simulink model "b6_formation2"  (R2021b)
settings: Solver=FixedStepAuto  StartTime=0.0  StopTime=inf  FixedStep=sampleTime  RelTol=1e-3
PreLoadFcn:
  | % Simulation parameters
  | %load exampleMap
  | 
  | % Lidar parameters
  | sensorOffset = [0,0];
  | scanAngles = -pi/2:pi/6:pi/2;
  | maxRange = 0.3;
InitFcn:
  | sampleTime = 0.05;
  | nMedianSize=3;
  | % Robot parameters
  | wheelRadius = 0.0335;
  | robotRadius = 0.8*0.116;
  | 
  | %角速度坐标
  | ks=1;
  | 
  | % Lidar parameters
  | sensorOffset = [0,0];
  | scanAngles = -pi:pi/36:pi;
  | maxRange = 0.2;
  | 
  | %车初始位置
  | init_pose_1=[1  1.3  pi/2]';
  | init_pose_2=[0.85 1  pi/2]';
  | init_pose_3=[1.15 1  pi/2]';
  | init_pose_4=[0.7  0.7 pi/2]';
  | init_pose_5=[1  0.7 pi/2]';
  | init_pose_6=[1.3 0.7  pi/2]';
  | 
  | %pp算法性能参数
  | Vd_pp=0.25;
  | Wd_pp=0.25*pi;
  | dist_pp=0.2;
  | GoalRadius=0.1;
  | numSector=72;
  | rangeDis=[0.03,maxRange];
  | thresholds=[0.03 0.1];
  | safetyDis=0.1;
  | minimumTurningRadius=0.2*0.2/3;
undefined symbols (not defined in the file): Angular, DiscIntNeverNeededParam, Linear, Pose, recovery_w, Twist
libraries: robotlib x42, dspstat3 x18, mobileRoboticsLib x7, robotmobilelib x6, robotalgslib x6
(part 4 of 5)

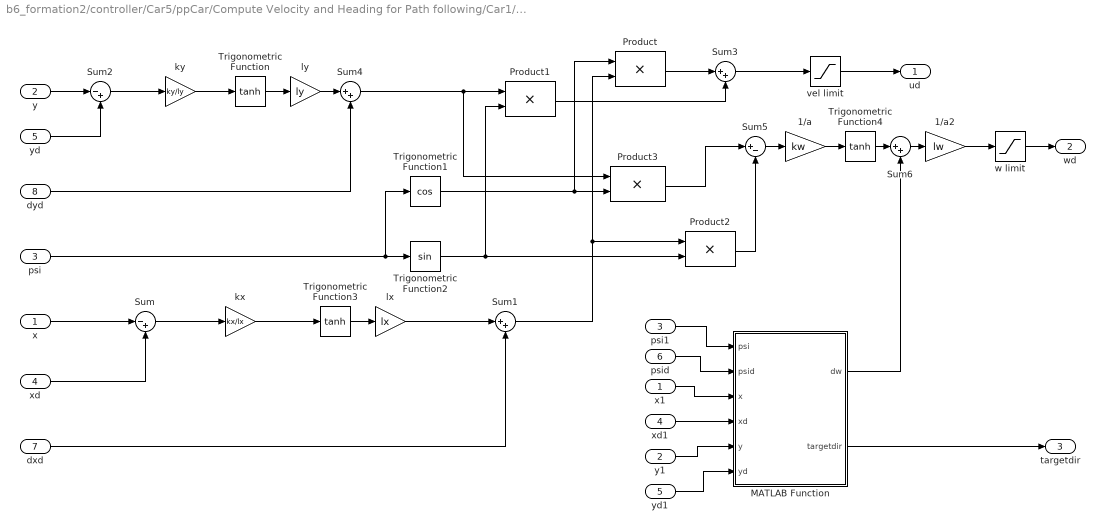
== system b6_formation2/controller/Car5/ppCar/Compute Velocity and Heading for Path following/Car1/Kinematicc Controller ==
  x : Inport
  y : Inport  Port=2
  psi : Inport  Port=3
  xd : Inport  Port=4
  yd : Inport  Port=5
  psid : Inport  Port=6
  dxd : Inport  Port=7
  dyd : Inport  Port=8
  1/a : Gain  Gain=kw  SaturateOnIntegerOverflow=on  OutDataTypeStr=Inherit: Same as input  ParamDataTypeStr=Inherit: Same as input
  1/a2 : Gain  Gain=lw  SaturateOnIntegerOverflow=on  OutDataTypeStr=Inherit: Same as input  ParamDataTypeStr=Inherit: Same as input
  MATLAB Function : MATLAB Function  TreatAsAtomicUnit=on
  Product{,1..3} (4 alike) : Product  SaturateOnIntegerOverflow=on  OutDataTypeStr=Inherit: Same as first input
  Sum : Sum  Inputs=|-+  SaturateOnIntegerOverflow=on
  Sum{1,3..4,6} (4 alike) : Sum  Inputs=|++  SaturateOnIntegerOverflow=on
  Sum2 : Sum  Inputs=|-+  SaturateOnIntegerOverflow=on
  Sum5 : Sum  Inputs=|+-  SaturateOnIntegerOverflow=on
  Trigonometric Function : Trigonometry  Operator=tanh
  Trigonometric Function1 : Trigonometry  Operator=cos
  Trigonometric Function2 : Trigonometry
  Trigonometric Function3 : Trigonometry  Operator=tanh
  Trigonometric Function4 : Trigonometry  Operator=tanh
  kx : Gain  Gain=kx/lx  SaturateOnIntegerOverflow=on  OutDataTypeStr=Inherit: Same as input  ParamDataTypeStr=Inherit: Same as input
  ky : Gain  Gain=ky/ly  SaturateOnIntegerOverflow=on  OutDataTypeStr=Inherit: Same as input  ParamDataTypeStr=Inherit: Same as input
  lx : Gain  Gain=lx  SaturateOnIntegerOverflow=on  OutDataTypeStr=Inherit: Same as input  ParamDataTypeStr=Inherit: Same as input
  ly : Gain  Gain=ly  SaturateOnIntegerOverflow=on  OutDataTypeStr=Inherit: Same as input  ParamDataTypeStr=Inherit: Same as input
  psi1 : InportShadow  Port=3
  vel limit : Saturate  UpperLimit=Vmax  LowerLimit=-0.2*Vmax
  w limit : Saturate  UpperLimit=Wmax  LowerLimit=-Wmax
  x1 : InportShadow
  xd1 : InportShadow  Port=4
  y1 : InportShadow  Port=2
  yd1 : InportShadow  Port=5
  ud : Outport
  wd : Outport  Port=2
  targetdir : Outport  Port=3
  wires:
  kx/1 -> Trigonometric Function3/1
  ky/1 -> Trigonometric Function/1
  Trigonometric Function1/1 -> Product3/2, Product/1
  Sum/1 -> kx/1
  y/1 -> Sum2/1
  Sum4/1 -> Product1/1, Product3/1
  Trigonometric Function2/1 -> Product2/2, Product1/2
  Sum3/1 -> vel limit/1
  dxd/1 -> Sum1/2
  dyd/1 -> Sum4/2
  ly/1 -> Sum4/1
  Trigonometric Function/1 -> ly/1
  lx/1 -> Sum1/1
  Trigonometric Function3/1 -> lx/1
  yd/1 -> Sum2/2
  xd/1 -> Sum/2
  x/1 -> Sum/1
  psi/1 -> Trigonometric Function2/1, Trigonometric Function1/1
  Sum1/1 -> Product2/1, Product/2
  Sum2/1 -> ky/1
  Product/1 -> Sum3/1
  Product1/1 -> Sum3/2
  Product3/1 -> Sum5/1
  Product2/1 -> Sum5/2
  Sum5/1 -> 1/a/1
  Trigonometric Function4/1 -> Sum6/1
  1/a/1 -> Trigonometric Function4/1
  vel limit/1 -> ud/1
  w limit/1 -> wd/1
  1/a2/1 -> w limit/1
  Sum6/1 -> 1/a2/1
  psid/1 -> MATLAB Function/2(psid)
  psi1/1 -> MATLAB Function/1(psi)
  x1/1 -> MATLAB Function/3(x)
  xd1/1 -> MATLAB Function/4(xd)
  y1/1 -> MATLAB Function/5(y)
  yd1/1 -> MATLAB Function/6(yd)
  MATLAB Function/1(dw) -> Sum6/2
  MATLAB Function/2(targetdir) -> targetdir/1

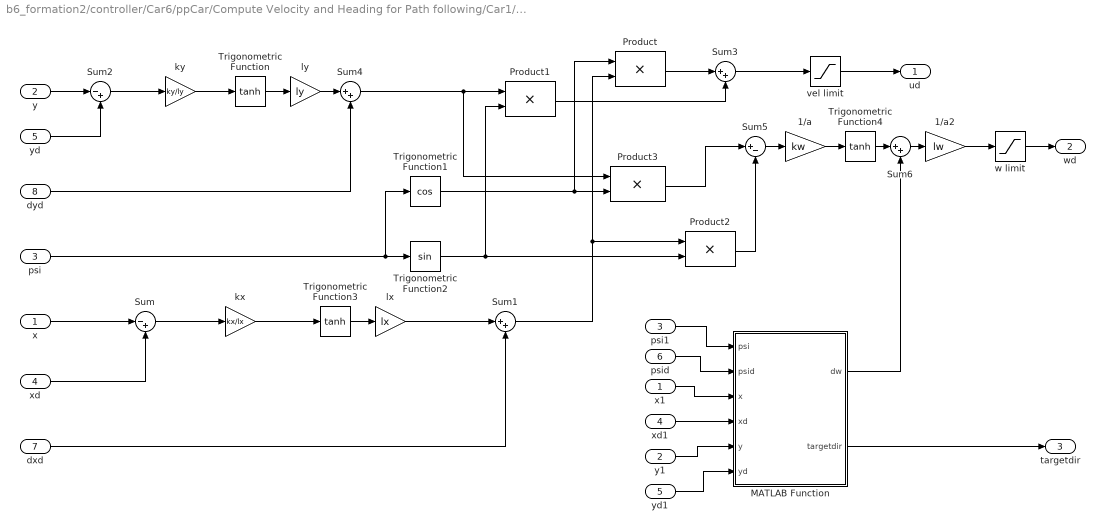
== system b6_formation2/controller/Car6/ppCar/Compute Velocity and Heading for Path following/Car1/Kinematicc Controller ==
  x : Inport
  y : Inport  Port=2
  psi : Inport  Port=3
  xd : Inport  Port=4
  yd : Inport  Port=5
  psid : Inport  Port=6
  dxd : Inport  Port=7
  dyd : Inport  Port=8
  1/a : Gain  Gain=kw  SaturateOnIntegerOverflow=on  OutDataTypeStr=Inherit: Same as input  ParamDataTypeStr=Inherit: Same as input
  1/a2 : Gain  Gain=lw  SaturateOnIntegerOverflow=on  OutDataTypeStr=Inherit: Same as input  ParamDataTypeStr=Inherit: Same as input
  MATLAB Function : MATLAB Function  TreatAsAtomicUnit=on
  Product{,1..3} (4 alike) : Product  SaturateOnIntegerOverflow=on  OutDataTypeStr=Inherit: Same as first input
  Sum : Sum  Inputs=|-+  SaturateOnIntegerOverflow=on
  Sum{1,3..4,6} (4 alike) : Sum  Inputs=|++  SaturateOnIntegerOverflow=on
  Sum2 : Sum  Inputs=|-+  SaturateOnIntegerOverflow=on
  Sum5 : Sum  Inputs=|+-  SaturateOnIntegerOverflow=on
  Trigonometric Function : Trigonometry  Operator=tanh
  Trigonometric Function1 : Trigonometry  Operator=cos
  Trigonometric Function2 : Trigonometry
  Trigonometric Function3 : Trigonometry  Operator=tanh
  Trigonometric Function4 : Trigonometry  Operator=tanh
  kx : Gain  Gain=kx/lx  SaturateOnIntegerOverflow=on  OutDataTypeStr=Inherit: Same as input  ParamDataTypeStr=Inherit: Same as input
  ky : Gain  Gain=ky/ly  SaturateOnIntegerOverflow=on  OutDataTypeStr=Inherit: Same as input  ParamDataTypeStr=Inherit: Same as input
  lx : Gain  Gain=lx  SaturateOnIntegerOverflow=on  OutDataTypeStr=Inherit: Same as input  ParamDataTypeStr=Inherit: Same as input
  ly : Gain  Gain=ly  SaturateOnIntegerOverflow=on  OutDataTypeStr=Inherit: Same as input  ParamDataTypeStr=Inherit: Same as input
  psi1 : InportShadow  Port=3
  vel limit : Saturate  UpperLimit=Vmax  LowerLimit=-0.2*Vmax
  w limit : Saturate  UpperLimit=Wmax  LowerLimit=-Wmax
  x1 : InportShadow
  xd1 : InportShadow  Port=4
  y1 : InportShadow  Port=2
  yd1 : InportShadow  Port=5
  ud : Outport
  wd : Outport  Port=2
  targetdir : Outport  Port=3
  wires:
  MATLAB Function/2(targetdir) -> targetdir/1
  MATLAB Function/1(dw) -> Sum6/2
  yd1/1 -> MATLAB Function/6(yd)
  y1/1 -> MATLAB Function/5(y)
  xd1/1 -> MATLAB Function/4(xd)
  x1/1 -> MATLAB Function/3(x)
  psi1/1 -> MATLAB Function/1(psi)
  psid/1 -> MATLAB Function/2(psid)
  Sum6/1 -> 1/a2/1
  1/a2/1 -> w limit/1
  w limit/1 -> wd/1
  vel limit/1 -> ud/1
  1/a/1 -> Trigonometric Function4/1
  Trigonometric Function4/1 -> Sum6/1
  Sum5/1 -> 1/a/1
  Product2/1 -> Sum5/2
  Product3/1 -> Sum5/1
  Product1/1 -> Sum3/2
  Product/1 -> Sum3/1
  Sum2/1 -> ky/1
  Sum1/1 -> Product/2, Product2/1
  psi/1 -> Trigonometric Function1/1, Trigonometric Function2/1
  x/1 -> Sum/1
  xd/1 -> Sum/2
  yd/1 -> Sum2/2
  Trigonometric Function3/1 -> lx/1
  lx/1 -> Sum1/1
  Trigonometric Function/1 -> ly/1
  ly/1 -> Sum4/1
  dyd/1 -> Sum4/2
  dxd/1 -> Sum1/2
  Sum3/1 -> vel limit/1
  Trigonometric Function2/1 -> Product1/2, Product2/2
  Sum4/1 -> Product3/1, Product1/1
  y/1 -> Sum2/1
  Sum/1 -> kx/1
  Trigonometric Function1/1 -> Product/1, Product3/2
  ky/1 -> Trigonometric Function/1
  kx/1 -> Trigonometric Function3/1

== matlab function b6_formation2/Subsystem/Car Pose Listener2/Subsystem/sensor2vCar4 ==
  data: V output; W output; VW_New input; VW_Msg input
function [V,W] = sensor2vCar(VW_New, VW_Msg)
persistent v0 w0
if isempty(v0)
    v0=0; 
    w0=0;    
end
if VW_New
    v0=VW_Msg.Linear.X;
    w0=VW_Msg.Angular.Z;
end

V=v0;
W=-w0;

== matlab function b6_formation2/controller/Car2/ppCar/Adjust Velocities to Avoid Obstacles/Path Following/Compute Angular Velocity ==
  data: steeringDir input; w output; wMax input
function w = exampleHelperComputeAngularVelocity(steeringDir, wMax)
%EXAMPLEHELPERCOMPUTEANGULARVELOCITY Compute angular velocity
%   W = exampleHelperComputeAngularVelocity(STEERINGDIR)
%   returns the angular velocity W for a differential drive robot in radians
%   per second for a given steering direction STEERINGDIR in the robot's
%   coordinate frame in radians.
%
%   W = exampleHelperComputeAngularVelocity(STEERINGDIR, WMAX)
%   returns the angular velocity W for a differential drive robot in radians
%   per second for a given steering direction STEERINGDIR in the robot's
%   coordinate frame in radians and maximum angular velocity WMAX in
%   radians per second. The output angular velocity is saturated based on
%   the WMAX.
%
%   Example:
%       
%       w = exampleHelperComputeAngularVelocity(0.2, 1);

% Copyright 2015 The MathWorks, Inc.

%#codegen
%#ok<*EMCA>

% Allow variable input arguments
if nargin == 1   
    wMax = inf;
end

validateattributes(steeringDir, {'double'},{'real'},...
    'exampleHelperComputeAngularVelocity', 'STEERINGDIR', 1);
validateattributes(wMax, {'double'},{'real', 'positive'},...
    'exampleHelperComputeAngularVelocity', 'WMAX', 2);

% Computing in robot's coordinate frame
curPose = [0 0 0];

% The following computation is similar to robotics.PurePursuit
lookaheadPoint = [cos(steeringDir), sin(steeringDir)];
slope = atan2((lookaheadPoint(2) - curPose(2)), ...
    (lookaheadPoint(1) - curPose(1)));
alpha = angdiff(curPose(3), slope);

% Angular velocity command for a differential drive robot is
% equal to the desired curvature to be followed by the robot.

% w = (2*sin(alpha));
% 
% % Pick a constant rotation when robot is facing in the opposite
% % direction of the path
% if abs(abs(alpha) - pi) < 1e-12
%     w = sign(w)*1;
% end
% % if abs(alpha)>pi/3
% %     w=sign(alpha)*wMax;
% % else
% %     w=0.3*alpha;
% % end
% 
% if abs(w) > wMax
%     w = sign(w)*wMax;
% end
w = sign(alpha)*wMax;

end

== matlab function b6_formation2/controller/Car2/ppCar/Compute Velocity and Heading for Path following/Car1/Kinematicc Controller/MATLAB Function ==
  data: psi input; dw output; psid input; x input; xd input; y input; yd input; targetdir output
function [dw,targetdir]= fcn(psi,psid,x,xd,y,yd)

if norm([xd-x,yd-y])<0.15    
    targetdir=angdiff(psi,psid);
    dw=tanh(targetdir);    
else
    dw=0;
    targetdir=angdiff(psi,atan2(yd-y,xd-x));
end

== matlab function b6_formation2/controller/Car1/ppCar/Adjust Velocities to Avoid Obstacles/Path Following/Compute Angular Velocity ==
  data: steeringDir input; w output; wMax input
function w = exampleHelperComputeAngularVelocity(steeringDir, wMax)
%EXAMPLEHELPERCOMPUTEANGULARVELOCITY Compute angular velocity
%   W = exampleHelperComputeAngularVelocity(STEERINGDIR)
%   returns the angular velocity W for a differential drive robot in radians
%   per second for a given steering direction STEERINGDIR in the robot's
%   coordinate frame in radians.
%
%   W = exampleHelperComputeAngularVelocity(STEERINGDIR, WMAX)
%   returns the angular velocity W for a differential drive robot in radians
%   per second for a given steering direction STEERINGDIR in the robot's
%   coordinate frame in radians and maximum angular velocity WMAX in
%   radians per second. The output angular velocity is saturated based on
%   the WMAX.
%
%   Example:
%       
%       w = exampleHelperComputeAngularVelocity(0.2, 1);

% Copyright 2015 The MathWorks, Inc.

%#codegen
%#ok<*EMCA>

% Allow variable input arguments
if nargin == 1   
    wMax = inf;
end

validateattributes(steeringDir, {'double'},{'real'},...
    'exampleHelperComputeAngularVelocity', 'STEERINGDIR', 1);
validateattributes(wMax, {'double'},{'real', 'positive'},...
    'exampleHelperComputeAngularVelocity', 'WMAX', 2);

% Computing in robot's coordinate frame
curPose = [0 0 0];

% The following computation is similar to robotics.PurePursuit
lookaheadPoint = [cos(steeringDir), sin(steeringDir)];
slope = atan2((lookaheadPoint(2) - curPose(2)), ...
    (lookaheadPoint(1) - curPose(1)));
alpha = angdiff(curPose(3), slope);

% Angular velocity command for a differential drive robot is
% equal to the desired curvature to be followed by the robot.

% w = (2*sin(alpha));
% 
% % Pick a constant rotation when robot is facing in the opposite
% % direction of the path
% if abs(abs(alpha) - pi) < 1e-12
%     w = sign(w)*1;
% end
% % if abs(alpha)>pi/3
% %     w=sign(alpha)*wMax;
% % else
% %     w=0.3*alpha;
% % end
% 
% if abs(w) > wMax
%     w = sign(w)*wMax;
% end
w = sign(alpha)*wMax;

end

== matlab function b6_formation2/controller/Car1/ppCar/Compute Velocity and Heading for Path following/Car1/Kinematicc Controller/MATLAB Function ==
  data: psi input; dw output; psid input; x input; xd input; y input; yd input; targetdir output
function [dw,targetdir]= fcn(psi,psid,x,xd,y,yd)

if norm([xd-x,yd-y])<0.15    
    targetdir=angdiff(psi,psid);
    dw=tanh(targetdir);    
else
    dw=0;
    targetdir=angdiff(psi,atan2(yd-y,xd-x));
end

== matlab function b6_formation2/ROS_simulation/ros1/MATLAB Function3 ==
  data: IsNew input; cmdMsg input; vref output; wref output
function [vref, wref] = ReadCMD(IsNew, cmdMsg)
persistent vref0 wref0
if isempty(vref0)
    vref0=0;
    wref0=0;
end
if IsNew
    vref0=cmdMsg.Linear.X;
    wref0=cmdMsg.Angular.Z;
end
vref=vref0;wref=wref0;

== matlab function b6_formation2/Subsystem/Car Pose Listener1/Subsystem/sensor2vCar ==
  data: x_init output; y_init output; yaw_init output; flag output; poseNew input; poseMsg input
function [x_init,y_init,yaw_init,flag] = sensor2vCar(poseNew, poseMsg)
persistent x0 y0 yaw0 yaw1 x0_init y0_init yaw0_init fStart
if isempty(x0)
    x0=-10; y0=-10; yaw0=0; yaw1=0;   
    x0_init=-10;y0_init=-10;yaw0_init=0;
    fStart=0;
end
if poseNew
    if x0==poseMsg.Pose.Pose.Position.X&&y0==poseMsg.Pose.Pose.Position.Y
        flag=1;
    else
        x0=poseMsg.Pose.Pose.Position.X;
        y0=poseMsg.Pose.Pose.Position.Y;   
        %yaw2=atan2(2*(poseMsg.Pose.Pose.Orientation.Z*poseMsg.Pose.Pose.Orientation.W),1-2*(poseMsg.Pose.Pose.Orientation.Z^2)); 
        eul=quat2eul([poseMsg.Pose.Pose.Orientation.W,poseMsg.Pose.Pose.Orientation.X,poseMsg.Pose.Pose.Orientation.Y,poseMsg.Pose.Pose.Orientation.Z]);
        yaw2=eul(1);
        %对前后角度差使用积分，恢复yaw的连续性
        yaw0=yaw0+angdiff(yaw1,yaw2);
        yaw1=yaw2;
        flag=0;        
        x0_init=x0;
        y0_init=y0;
        yaw0_init=yaw0;
        fStart=1;
    end 
else
    if fStart
        flag=1;
    else
        flag=0;
    end
end

x_init=x0_init;y_init=y0_init;yaw_init=yaw0_init;

== matlab function b6_formation2/controller/Car3/ppCar/Adjust Velocities to Avoid Obstacles/Path Following/Compute Angular Velocity ==
  data: steeringDir input; w output; wMax input
function w = exampleHelperComputeAngularVelocity(steeringDir, wMax)
%EXAMPLEHELPERCOMPUTEANGULARVELOCITY Compute angular velocity
%   W = exampleHelperComputeAngularVelocity(STEERINGDIR)
%   returns the angular velocity W for a differential drive robot in radians
%   per second for a given steering direction STEERINGDIR in the robot's
%   coordinate frame in radians.
%
%   W = exampleHelperComputeAngularVelocity(STEERINGDIR, WMAX)
%   returns the angular velocity W for a differential drive robot in radians
%   per second for a given steering direction STEERINGDIR in the robot's
%   coordinate frame in radians and maximum angular velocity WMAX in
%   radians per second. The output angular velocity is saturated based on
%   the WMAX.
%
%   Example:
%       
%       w = exampleHelperComputeAngularVelocity(0.2, 1);

% Copyright 2015 The MathWorks, Inc.

%#codegen
%#ok<*EMCA>

% Allow variable input arguments
if nargin == 1   
    wMax = inf;
end

validateattributes(steeringDir, {'double'},{'real'},...
    'exampleHelperComputeAngularVelocity', 'STEERINGDIR', 1);
validateattributes(wMax, {'double'},{'real', 'positive'},...
    'exampleHelperComputeAngularVelocity', 'WMAX', 2);

% Computing in robot's coordinate frame
curPose = [0 0 0];

% The following computation is similar to robotics.PurePursuit
lookaheadPoint = [cos(steeringDir), sin(steeringDir)];
slope = atan2((lookaheadPoint(2) - curPose(2)), ...
    (lookaheadPoint(1) - curPose(1)));
alpha = angdiff(curPose(3), slope);

% Angular velocity command for a differential drive robot is
% equal to the desired curvature to be followed by the robot.

% w = (2*sin(alpha));
% 
% % Pick a constant rotation when robot is facing in the opposite
% % direction of the path
% if abs(abs(alpha) - pi) < 1e-12
%     w = sign(w)*1;
% end
% % if abs(alpha)>pi/3
% %     w=sign(alpha)*wMax;
% % else
% %     w=0.3*alpha;
% % end
% 
% if abs(w) > wMax
%     w = sign(w)*wMax;
% end
w = sign(alpha)*wMax;

end

== matlab function b6_formation2/controller/Car3/ppCar/Compute Velocity and Heading for Path following/Car1/Kinematicc Controller/MATLAB Function ==
  data: psi input; dw output; psid input; x input; xd input; y input; yd input; targetdir output
function [dw,targetdir]= fcn(psi,psid,x,xd,y,yd)

if norm([xd-x,yd-y])<0.15    
    targetdir=angdiff(psi,psid);
    dw=tanh(targetdir);    
else
    dw=0;
    targetdir=angdiff(psi,atan2(yd-y,xd-x));
end

== matlab function b6_formation2/Subsystem/Car Pose Listener/Subsystem/sensor2vCar4 ==
  data: V output; W output; VW_New input; VW_Msg input
function [V,W] = sensor2vCar(VW_New, VW_Msg)
persistent v0 w0
if isempty(v0)
    v0=0; 
    w0=0;    
end
if VW_New
    v0=VW_Msg.Linear.X;
    w0=VW_Msg.Angular.Z;
end

V=v0;
W=-w0;

== matlab function b6_formation2/ROS_simulation/ros2/MATLAB Function3 ==
  data: IsNew input; cmdMsg input; vref output; wref output
function [vref, wref] = ReadCMD(IsNew, cmdMsg)
persistent vref0 wref0
if isempty(vref0)
    vref0=0;
    wref0=0;
end
if IsNew
    vref0=cmdMsg.Linear.X;
    wref0=cmdMsg.Angular.Z;
end
vref=vref0;wref=wref0;

== matlab function b6_formation2/ROS_simulation/ros3/MATLAB Function3 ==
  data: IsNew input; cmdMsg input; vref output; wref output
function [vref, wref] = ReadCMD(IsNew, cmdMsg)
persistent vref0 wref0
if isempty(vref0)
    vref0=0;
    wref0=0;
end
if IsNew
    vref0=cmdMsg.Linear.X;
    wref0=cmdMsg.Angular.Z;
end
vref=vref0;wref=wref0;

== matlab function b6_formation2/ROS_simulation/ros4/MATLAB Function3 ==
  data: IsNew input; cmdMsg input; vref output; wref output
function [vref, wref] = ReadCMD(IsNew, cmdMsg)
persistent vref0 wref0
if isempty(vref0)
    vref0=0;
    wref0=0;
end
if IsNew
    vref0=cmdMsg.Linear.X;
    wref0=cmdMsg.Angular.Z;
end
vref=vref0;wref=wref0;

== matlab function b6_formation2/controller/Car4/ppCar/Adjust Velocities to Avoid Obstacles/Path Following/Compute Angular Velocity ==
  data: steeringDir input; w output; wMax input
function w = exampleHelperComputeAngularVelocity(steeringDir, wMax)
%EXAMPLEHELPERCOMPUTEANGULARVELOCITY Compute angular velocity
%   W = exampleHelperComputeAngularVelocity(STEERINGDIR)
%   returns the angular velocity W for a differential drive robot in radians
%   per second for a given steering direction STEERINGDIR in the robot's
%   coordinate frame in radians.
%
%   W = exampleHelperComputeAngularVelocity(STEERINGDIR, WMAX)
%   returns the angular velocity W for a differential drive robot in radians
%   per second for a given steering direction STEERINGDIR in the robot's
%   coordinate frame in radians and maximum angular velocity WMAX in
%   radians per second. The output angular velocity is saturated based on
%   the WMAX.
%
%   Example:
%       
%       w = exampleHelperComputeAngularVelocity(0.2, 1);

% Copyright 2015 The MathWorks, Inc.

%#codegen
%#ok<*EMCA>

% Allow variable input arguments
if nargin == 1   
    wMax = inf;
end

validateattributes(steeringDir, {'double'},{'real'},...
    'exampleHelperComputeAngularVelocity', 'STEERINGDIR', 1);
validateattributes(wMax, {'double'},{'real', 'positive'},...
    'exampleHelperComputeAngularVelocity', 'WMAX', 2);

% Computing in robot's coordinate frame
curPose = [0 0 0];

% The following computation is similar to robotics.PurePursuit
lookaheadPoint = [cos(steeringDir), sin(steeringDir)];
slope = atan2((lookaheadPoint(2) - curPose(2)), ...
    (lookaheadPoint(1) - curPose(1)));
alpha = angdiff(curPose(3), slope);

% Angular velocity command for a differential drive robot is
% equal to the desired curvature to be followed by the robot.

% w = (2*sin(alpha));
% 
% % Pick a constant rotation when robot is facing in the opposite
% % direction of the path
% if abs(abs(alpha) - pi) < 1e-12
%     w = sign(w)*1;
% end
% % if abs(alpha)>pi/3
% %     w=sign(alpha)*wMax;
% % else
% %     w=0.3*alpha;
% % end
% 
% if abs(w) > wMax
%     w = sign(w)*wMax;
% end
w = sign(alpha)*wMax;

end

== matlab function b6_formation2/controller/Car4/ppCar/Compute Velocity and Heading for Path following/Car1/Kinematicc Controller/MATLAB Function ==
  data: psi input; dw output; psid input; x input; xd input; y input; yd input; targetdir output
function [dw,targetdir]= fcn(psi,psid,x,xd,y,yd)

if norm([xd-x,yd-y])<0.15    
    targetdir=angdiff(psi,psid);
    dw=tanh(targetdir);    
else
    dw=0;
    targetdir=angdiff(psi,atan2(yd-y,xd-x));
end

== matlab function b6_formation2/controller/Car5/ppCar/Adjust Velocities to Avoid Obstacles/Path Following/Compute Angular Velocity ==
  data: steeringDir input; w output; wMax input
function w = exampleHelperComputeAngularVelocity(steeringDir, wMax)
%EXAMPLEHELPERCOMPUTEANGULARVELOCITY Compute angular velocity
%   W = exampleHelperComputeAngularVelocity(STEERINGDIR)
%   returns the angular velocity W for a differential drive robot in radians
%   per second for a given steering direction STEERINGDIR in the robot's
%   coordinate frame in radians.
%
%   W = exampleHelperComputeAngularVelocity(STEERINGDIR, WMAX)
%   returns the angular velocity W for a differential drive robot in radians
%   per second for a given steering direction STEERINGDIR in the robot's
%   coordinate frame in radians and maximum angular velocity WMAX in
%   radians per second. The output angular velocity is saturated based on
%   the WMAX.
%
%   Example:
%       
%       w = exampleHelperComputeAngularVelocity(0.2, 1);

% Copyright 2015 The MathWorks, Inc.

%#codegen
%#ok<*EMCA>

% Allow variable input arguments
if nargin == 1   
    wMax = inf;
end

validateattributes(steeringDir, {'double'},{'real'},...
    'exampleHelperComputeAngularVelocity', 'STEERINGDIR', 1);
validateattributes(wMax, {'double'},{'real', 'positive'},...
    'exampleHelperComputeAngularVelocity', 'WMAX', 2);

% Computing in robot's coordinate frame
curPose = [0 0 0];

% The following computation is similar to robotics.PurePursuit
lookaheadPoint = [cos(steeringDir), sin(steeringDir)];
slope = atan2((lookaheadPoint(2) - curPose(2)), ...
    (lookaheadPoint(1) - curPose(1)));
alpha = angdiff(curPose(3), slope);

% Angular velocity command for a differential drive robot is
% equal to the desired curvature to be followed by the robot.

% w = (2*sin(alpha));
% 
% % Pick a constant rotation when robot is facing in the opposite
% % direction of the path
% if abs(abs(alpha) - pi) < 1e-12
%     w = sign(w)*1;
% end
% % if abs(alpha)>pi/3
% %     w=sign(alpha)*wMax;
% % else
% %     w=0.3*alpha;
% % end
% 
% if abs(w) > wMax
%     w = sign(w)*wMax;
% end
w = sign(alpha)*wMax;

end

== matlab function b6_formation2/ROS_simulation/ros1/MATLAB Function ==
  data: yaw input; x output; y output; z output; w output
function [x,y,z,w]=ToQuaternion(yaw)
%https://blog.csdn.net/xiaoma_bk/article/details/79082629
pitch=0;
roll=0;

   cy = cos(yaw * 0.5);
    sy = sin(yaw * 0.5);
    cp = cos(pitch * 0.5);
    sp = sin(pitch * 0.5);
    cr = cos(roll * 0.5);
    sr = sin(roll * 0.5);
 

   w = cy * cp * cr + sy * sp * sr;
   x = cy * cp * sr - sy * sp * cr;
   y = sy * cp * sr + cy * sp * cr;
    z = sy * cp * cr - cy * sp * sr;

== matlab function b6_formation2/ROS_simulation/ros2/MATLAB Function ==
  data: yaw input; x output; y output; z output; w output
function [x,y,z,w]=ToQuaternion(yaw)
%https://blog.csdn.net/xiaoma_bk/article/details/79082629
pitch=0;
roll=0;

   cy = cos(yaw * 0.5);
    sy = sin(yaw * 0.5);
    cp = cos(pitch * 0.5);
    sp = sin(pitch * 0.5);
    cr = cos(roll * 0.5);
    sr = sin(roll * 0.5);
 

   w = cy * cp * cr + sy * sp * sr;
   x = cy * cp * sr - sy * sp * cr;
   y = sy * cp * sr + cy * sp * cr;
    z = sy * cp * cr - cy * sp * sr;

== matlab function b6_formation2/ROS_simulation/ros3/MATLAB Function ==
  data: yaw input; x output; y output; z output; w output
function [x,y,z,w]=ToQuaternion(yaw)
%https://blog.csdn.net/xiaoma_bk/article/details/79082629
pitch=0;
roll=0;

   cy = cos(yaw * 0.5);
    sy = sin(yaw * 0.5);
    cp = cos(pitch * 0.5);
    sp = sin(pitch * 0.5);
    cr = cos(roll * 0.5);
    sr = sin(roll * 0.5);
 

   w = cy * cp * cr + sy * sp * sr;
   x = cy * cp * sr - sy * sp * cr;
   y = sy * cp * sr + cy * sp * cr;
    z = sy * cp * cr - cy * sp * sr;

== matlab function b6_formation2/ROS_simulation/ros4/MATLAB Function ==
  data: yaw input; x output; y output; z output; w output
function [x,y,z,w]=ToQuaternion(yaw)
%https://blog.csdn.net/xiaoma_bk/article/details/79082629
pitch=0;
roll=0;

   cy = cos(yaw * 0.5);
    sy = sin(yaw * 0.5);
    cp = cos(pitch * 0.5);
    sp = sin(pitch * 0.5);
    cr = cos(roll * 0.5);
    sr = sin(roll * 0.5);
 

   w = cy * cp * cr + sy * sp * sr;
   x = cy * cp * sr - sy * sp * cr;
   y = sy * cp * sr + cy * sp * cr;
    z = sy * cp * cr - cy * sp * sr;

== matlab function b6_formation2/ROS_simulation/ros5/MATLAB Function ==
  data: yaw input; x output; y output; z output; w output
function [x,y,z,w]=ToQuaternion(yaw)
%https://blog.csdn.net/xiaoma_bk/article/details/79082629
pitch=0;
roll=0;

   cy = cos(yaw * 0.5);
    sy = sin(yaw * 0.5);
    cp = cos(pitch * 0.5);
    sp = sin(pitch * 0.5);
    cr = cos(roll * 0.5);
    sr = sin(roll * 0.5);
 

   w = cy * cp * cr + sy * sp * sr;
   x = cy * cp * sr - sy * sp * cr;
   y = sy * cp * sr + cy * sp * cr;
    z = sy * cp * cr - cy * sp * sr;

== matlab function b6_formation2/ROS_simulation/ros6/MATLAB Function ==
  data: yaw input; x output; y output; z output; w output
function [x,y,z,w]=ToQuaternion(yaw)
%https://blog.csdn.net/xiaoma_bk/article/details/79082629
pitch=0;
roll=0;

   cy = cos(yaw * 0.5);
    sy = sin(yaw * 0.5);
    cp = cos(pitch * 0.5);
    sp = sin(pitch * 0.5);
    cr = cos(roll * 0.5);
    sr = sin(roll * 0.5);
 

   w = cy * cp * cr + sy * sp * sr;
   x = cy * cp * sr - sy * sp * cr;
   y = sy * cp * sr + cy * sp * cr;
    z = sy * cp * cr - cy * sp * sr;

== matlab function b6_formation2/ROS_simulation/ros5/MATLAB Function3 ==
  data: IsNew input; cmdMsg input; vref output; wref output
function [vref, wref] = ReadCMD(IsNew, cmdMsg)
persistent vref0 wref0
if isempty(vref0)
    vref0=0;
    wref0=0;
end
if IsNew
    vref0=cmdMsg.Linear.X;
    wref0=cmdMsg.Angular.Z;
end
vref=vref0;wref=wref0;

== matlab function b6_formation2/ROS_simulation/ros6/MATLAB Function3 ==
  data: IsNew input; cmdMsg input; vref output; wref output
function [vref, wref] = ReadCMD(IsNew, cmdMsg)
persistent vref0 wref0
if isempty(vref0)
    vref0=0;
    wref0=0;
end
if IsNew
    vref0=cmdMsg.Linear.X;
    wref0=cmdMsg.Angular.Z;
end
vref=vref0;wref=wref0;

== matlab function b6_formation2/controller/Car5/ppCar/Compute Velocity and Heading for Path following/Car1/Kinematicc Controller/MATLAB Function ==
  data: psi input; dw output; psid input; x input; xd input; y input; yd input; targetdir output
function [dw,targetdir]= fcn(psi,psid,x,xd,y,yd)

if norm([xd-x,yd-y])<0.15    
    targetdir=angdiff(psi,psid);
    dw=tanh(targetdir);    
else
    dw=0;
    targetdir=angdiff(psi,atan2(yd-y,xd-x));
end

== matlab function b6_formation2/controller/Car6/ppCar/Adjust Velocities to Avoid Obstacles/Path Following/Compute Angular Velocity ==
  data: steeringDir input; w output; wMax input
function w = exampleHelperComputeAngularVelocity(steeringDir, wMax)
%EXAMPLEHELPERCOMPUTEANGULARVELOCITY Compute angular velocity
%   W = exampleHelperComputeAngularVelocity(STEERINGDIR)
%   returns the angular velocity W for a differential drive robot in radians
%   per second for a given steering direction STEERINGDIR in the robot's
%   coordinate frame in radians.
%
%   W = exampleHelperComputeAngularVelocity(STEERINGDIR, WMAX)
%   returns the angular velocity W for a differential drive robot in radians
%   per second for a given steering direction STEERINGDIR in the robot's
%   coordinate frame in radians and maximum angular velocity WMAX in
%   radians per second. The output angular velocity is saturated based on
%   the WMAX.
%
%   Example:
%       
%       w = exampleHelperComputeAngularVelocity(0.2, 1);

% Copyright 2015 The MathWorks, Inc.

%#codegen
%#ok<*EMCA>

% Allow variable input arguments
if nargin == 1   
    wMax = inf;
end

validateattributes(steeringDir, {'double'},{'real'},...
    'exampleHelperComputeAngularVelocity', 'STEERINGDIR', 1);
validateattributes(wMax, {'double'},{'real', 'positive'},...
    'exampleHelperComputeAngularVelocity', 'WMAX', 2);

% Computing in robot's coordinate frame
curPose = [0 0 0];

% The following computation is similar to robotics.PurePursuit
lookaheadPoint = [cos(steeringDir), sin(steeringDir)];
slope = atan2((lookaheadPoint(2) - curPose(2)), ...
    (lookaheadPoint(1) - curPose(1)));
alpha = angdiff(curPose(3), slope);

% Angular velocity command for a differential drive robot is
% equal to the desired curvature to be followed by the robot.

% w = (2*sin(alpha));
% 
% % Pick a constant rotation when robot is facing in the opposite
% % direction of the path
% if abs(abs(alpha) - pi) < 1e-12
%     w = sign(w)*1;
% end
% % if abs(alpha)>pi/3
% %     w=sign(alpha)*wMax;
% % else
% %     w=0.3*alpha;
% % end
% 
% if abs(w) > wMax
%     w = sign(w)*wMax;
% end
w = sign(alpha)*wMax;

end

== matlab function b6_formation2/Subsystem/Car Pose Listener3/Subsystem/sensor2vCar ==
  data: x_init output; y_init output; yaw_init output; flag output; poseNew input; poseMsg input
function [x_init,y_init,yaw_init,flag] = sensor2vCar(poseNew, poseMsg)
persistent x0 y0 yaw0 yaw1 x0_init y0_init yaw0_init fStart
if isempty(x0)
    x0=-10; y0=-10; yaw0=0; yaw1=0;   
    x0_init=-10;y0_init=-10;yaw0_init=0;
    fStart=0;
end
if poseNew
    if x0==poseMsg.Pose.Pose.Position.X&&y0==poseMsg.Pose.Pose.Position.Y
        flag=1;
    else
        x0=poseMsg.Pose.Pose.Position.X;
        y0=poseMsg.Pose.Pose.Position.Y;   
        %yaw2=atan2(2*(poseMsg.Pose.Pose.Orientation.Z*poseMsg.Pose.Pose.Orientation.W),1-2*(poseMsg.Pose.Pose.Orientation.Z^2)); 
        eul=quat2eul([poseMsg.Pose.Pose.Orientation.W,poseMsg.Pose.Pose.Orientation.X,poseMsg.Pose.Pose.Orientation.Y,poseMsg.Pose.Pose.Orientation.Z]);
        yaw2=eul(1);
        %对前后角度差使用积分，恢复yaw的连续性
        yaw0=yaw0+angdiff(yaw1,yaw2);
        yaw1=yaw2;
        flag=0;        
        x0_init=x0;
        y0_init=y0;
        yaw0_init=yaw0;
        fStart=1;
    end 
else
    if fStart
        flag=1;
    else
        flag=0;
    end
end

x_init=x0_init;y_init=y0_init;yaw_init=yaw0_init;

== matlab function b6_formation2/controller/controller1/MATLAB Function1 ==
  data: poses input; idx input; ranges output; maxRange parameter; scanAngles parameter; robotRadius parameter

function ranges = genLidarSensor(poses,idx, maxRange, scanAngles, robotRadius)
%模拟激光雷达计算地图中障碍物距离

%计算部分
map=occupancyMap(3,3,50);
num=length(poses(1,:));%机器人总数
worldOffset=[0.5,0.5];%将世界坐标系偏移进地图
safetyDis=maxRange;
poseX=[poses(1,:)+worldOffset(1);poses(2,:)+worldOffset(2);poses(3,:)];
% for i=[1:idx-1 idx+1:num]
%     if poseX(i,1)>=0&&poseX(i,1)<=3&&poseX(i,2)>=0&&poseX(i,2)<=3        
%         setOccupancy(map,poseX(1:2,i)',1);
%     end
% end
obstacles = poseX(1:2,[1:idx-1 idx+1:num])';
setOccupancy(map,obstacles,ones(length(obstacles),1));
inflate(map,robotRadius);

if poseX(1,idx)>=0&&poseX(1,idx)<=3&&poseX(2,idx)>=0&&poseX(2,idx)<=3 
    vehiclePose = poseX(:,idx)';
    intsectionPts = rayIntersection(map,vehiclePose,scanAngles,safetyDis,0.7);
    offsets=intsectionPts-ones(length(scanAngles),1)*vehiclePose(1:2);
    ranges = sqrt(sum(offsets.^2,2));    
else
    ranges = nan(length(scanAngles),1);   
end

== matlab function b6_formation2/controller/Car6/ppCar/Compute Velocity and Heading for Path following/Car1/Kinematicc Controller/MATLAB Function ==
  data: psi input; dw output; psid input; x input; xd input; y input; yd input; targetdir output
function [dw,targetdir]= fcn(psi,psid,x,xd,y,yd)

if norm([xd-x,yd-y])<0.15    
    targetdir=angdiff(psi,psid);
    dw=tanh(targetdir);    
else
    dw=0;
    targetdir=angdiff(psi,atan2(yd-y,xd-x));
end

== matlab function b6_formation2/controller/controller1/MATLAB Function5 ==
  data: poses input; idx input; ranges output; maxRange parameter; scanAngles parameter; robotRadius parameter

function ranges = genLidarSensor(poses,idx, maxRange, scanAngles, robotRadius)
%模拟激光雷达计算地图中障碍物距离

%计算部分
map=occupancyMap(3,3,50);
num=length(poses(1,:));%机器人总数
worldOffset=[0.5,0.5];%将世界坐标系偏移进地图
safetyDis=maxRange;
poseX=[poses(1,:)+worldOffset(1);poses(2,:)+worldOffset(2);poses(3,:)];
% for i=[1:idx-1 idx+1:num]
%     if poseX(i,1)>=0&&poseX(i,1)<=3&&poseX(i,2)>=0&&poseX(i,2)<=3        
%         setOccupancy(map,poseX(1:2,i)',1);
%     end
% end
obstacles = poseX(1:2,[1:idx-1 idx+1:num])';
setOccupancy(map,obstacles,ones(length(obstacles),1));
inflate(map,robotRadius);

if poseX(1,idx)>=0&&poseX(1,idx)<=3&&poseX(2,idx)>=0&&poseX(2,idx)<=3 
    vehiclePose = poseX(:,idx)';
    intsectionPts = rayIntersection(map,vehiclePose,scanAngles,safetyDis,0.7);
    offsets=intsectionPts-ones(length(scanAngles),1)*vehiclePose(1:2);
    ranges = sqrt(sum(offsets.^2,2));    
else
    ranges = nan(length(scanAngles),1);   
end

== matlab function b6_formation2/Subsystem/Car Pose Listener3/Subsystem/sensor2vCar4 ==
  data: V output; W output; VW_New input; VW_Msg input
function [V,W] = sensor2vCar(VW_New, VW_Msg)
persistent v0 w0
if isempty(v0)
    v0=0; 
    w0=0;    
end
if VW_New
    v0=VW_Msg.Linear.X;
    w0=VW_Msg.Angular.Z;
end

V=v0;
W=-w0;
